simulink model "hexa_tilted_ANSFT"  (R2023a)
settings: Solver=ode1  StartTime=0.0  StopTime=tf  FixedStep=0.01  RelTol=1e-3
model workspace (MAT data in the model file):
  hover_2m = [0  0  0  0  0  0; 0  0  0  0  0  0; 2  2  2  2  2  2; 0  0  0  0  0  0; 0  0  0  0  0  0; 0  0  0  0  0  0]
  square = [0  0  0  0  0  0; 0  0  0  0  0  0; 2.5  2.5  2.5  2.5  2.5  0; 0  0  0  0  0  0; 0  0  0  0  0  0; 0  0  0  0  0  0]
  tf = Simulink.Parameter
  tf.Value = 60
  tf.DataType = 'auto'
  tf.Complexity = 'real'
  tf.Dimensions = [1 1]
  tray0 = [0  0  0  0  0  0; 0  0  0  0  0  0; 0  5  5  5  5  0; 0  0  0  0  0  0; 0  0  0  0  0  0; 0  0  0  0  0  0]
  tray1 = [0  0  0  0  0  0; 0  0  0  0  0  0; 0  5  2.5  5  2.5  0; 0  0  0  0  0  0; 0  0  0  0  0  0; 0  0  0  0  0  0]
  tray2 = [0  2  2  -2  -2  0; 0  0  -2  -2  2  0; 0  5  2.5  5  2.5  0; 0  0  0  0  0  0; 0  0  0  0  0  0; 0  0  0  0  0  0]
  tray3 = [0  2  2  -2  -2  0; 0  0  -2  -2  2  0; 0  5  2.5  5  2.5  0; 0  0  0  0  0  0; 0  0  0  0  0  0; 0  0  0.785  1.57  0.785  0]
  tray4 = [0  2  2  -2  -2  0; 0  0  -2  -2  2  0; 0  5  2.5  5  2.5  0; 0  0.15  0.15  0.15  0.15  0; 0  0  0  0  0  0; 0  0  0.785  1.57  0.785  0]
  tray5 = [0  0  0  0  0  0; 0  0  0  0  0  0; 0  5  2.5  5  2.5  0; 0  0.15  0.15  0  0  0; 0  0  0.15  0.15  0  0; 0  0  0  0  0  0]
  tray_yaw = [0  0  0  0  0  0; 0  0  0  0  0  0; 0  5  2.5  5  2.5  0; 0  0  0  0  0  0; 0  0  0  0  0  0; 0  0  0.785  1.57  0.785  0]
values from neighbouring files (symbols this model uses):
  F = [fx; fy; fz; tx; ty; tz]    [dump_quad_formulas.m]
undefined symbols (not defined in the file or in its folder): Light, MIL, sigbuilder_block
libraries: SignalEditorBlockLib x2, robotcorelib x1, sharedtransform x1, aerolibwind2 x1
settings Model: Creator=adan  LastModifiedBy=Adan Daniel
settings OptimizationCC: DefaultParameterBehavior=Inlined  EnhancedBackFolding=on  PassReuseOutputArgsAs=Individual arguments  ZeroExternalMemoryAtStartup=off  ZeroInternalMemoryAtStartup=off  OptimizeBlockOrder=speed  DifferentSizesBufferReuse=on  OptimizationCustomize=off  EfficientTunableParamExpr=on
settings DebuggingCC: ParameterTunabilityLossMsg=error
settings SFSimCC: MATLABDynamicMemAlloc=off
settings RTWCC: Description=Embedded Coder  SystemTargetFile=ert.tlc  TemplateMakefile=ert_default_tmf
settings CodeAppCC: ForceParamTrailComments=on  IgnoreCustomStorageClasses=off  OperatorAnnotations=on  SimulinkDataObjDesc=on  SFDataObjDesc=on  InsertBlockDesc=on
settings ERTTargetCC: TargetLangStandard=C99 (ISO)  GenerateSampleERTMain=on  InlinedParameterPlacement=NonHierarchical  ERTCustomFileTemplate=example_file_process.tlc

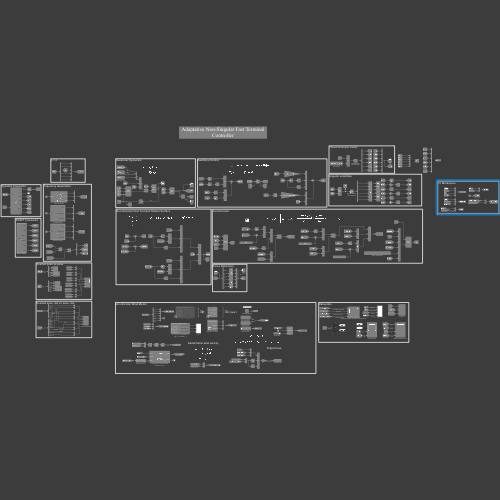
[thumbnail: Simulink's stored preview of the top-level diagram]
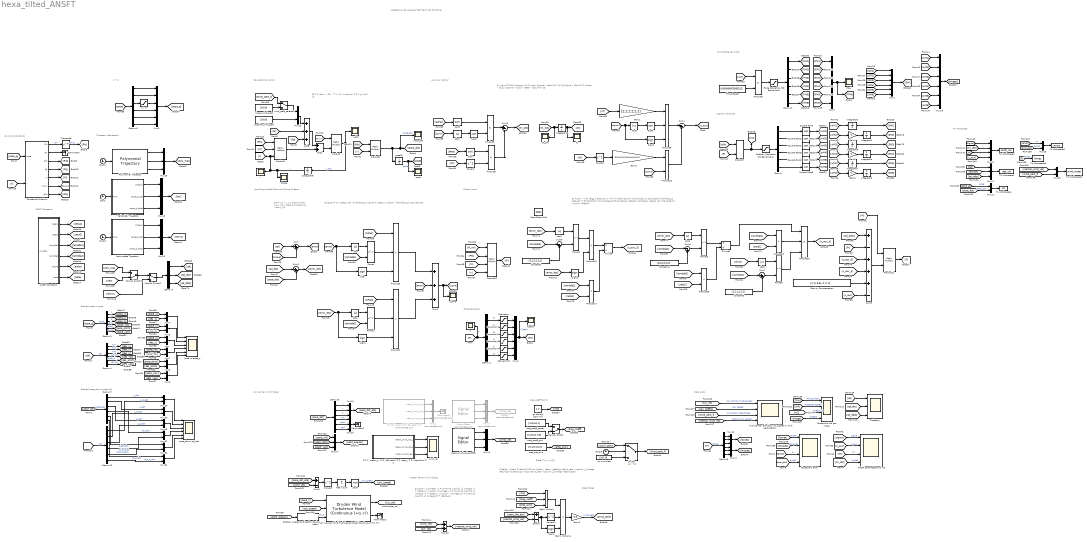
== system hexa_tilted_ANSFT ==
  note: To Workspace
  note: Von Kármán Wind Model
  note: $\Delta _ {\eta} = \frac{1}{2}\rho \alpha _ \eta A _\eta\big (\dot d_\eta - \upsilon _{\omega \eta}\big)^2\text{sign }\big (\dot d_\eta - \upsilon _{\omega \eta}\big)$$
  note: drag coeff from []
  note: $\upsilon _{\omega x} = \overline \upsilon _{ \omega x} + \delta_u \\ \upsilon _{\omega y} = \overline \upsilon _{ \omega y} + \delta_u \\ \upsilon _{\omega z} = \overline \upsilon _{ \omega z} + \delta_u$
  note: Auxiliary Control
  note: Non-Singular Fast Terminal Sliding Surface
  note: Control Input
  note: $e = x_d - x_1 \\ \dot e = \dot x_d - x_2 \\ \ddot e = \ddot x_d - \dot x_2$
  note: z > 0
  note: Adaptative Non-Singular Fast Terminal Controller
  note: ANSFT Constants
  note: Desired pose vs pose
  note: Trajectory Generation
  note: Dynamic Constants
  note: Data plots
  note: Angular velocities
  note: Thrust force per motor
  note: Hexarotor Dynamics
  note: Force Saturation
  note: $u = g(x) ^{-1} \Bigg [ \ddot \chi_d - f(x) + \frac{|\dot e|^{2-\lambda_2} sign(\dot e)}{\lambda_2 \zeta_2} + \frac{|\dot e|^{2-\lambda_2}}{\lambda_2 \zeta_2} \lambda_1 \zeta_1 |e|^{\lambda-1} - u_{aux} \Bigg ]$
  note: $\sigma = e + \zeta_1 |e| ^{\lambda_1} sign(e) + \zeta_2 | \dot e| ^{\lambda_2} sign(\dot e)$
  note: $u_{aux}=-2K(t) |\sigma|^{1/2} sign (\sigma) - \frac{K(t)^2}{2}\sigma \\ \dot K(t) = \alpha ^{1/2} |\sigma| ^{1/2} - \beta ^{1/2}K(t)^2$
  note: $F = M \dot v - \Phi ^T (v) Mv \\ \dot \chi = R^i_b (\chi) v$
  note: $\eta = \{x,y,z\}$
  note: Drag Forces
  note: Inertial frame wind velocity
  note: Desired pose_dot vs pose_dot
  ANSFT Constants : MATLAB Function  TreatAsAtomicUnit=on
  ANSFT parameters and vel : Scope  NumInputPorts=4
  Abs{,1..6} (7 alike) : Abs  SaturateOnIntegerOverflow=off
  Add2 : Sum
  Add5 : Sum  Inputs=+++
  Clock{,1..3} (4 alike) : Clock
  Constant2 : Constant  Value=[2;2;2;2;2;2]
  Constant3 : Constant  Value=[1;1;1;1;1;1]
  Constant4 : Constant  Value=[2;2;2;2;2;2]
  Constants Functions : MATLAB Function  TreatAsAtomicUnit=on
  Demux{,1..6,8..10} (10 alike) : Demux  Outputs=6
  Demux7 : Demux  Outputs=3
  Divide : Product  Inputs=*/
  Divide1 : Product  Inputs=*/
  F : Scope
  F_satur : Scope
  Force Saturation (RC Benchmark) : Saturate  UpperLimit=10  LowerLimit=0
  Forces and Vel per motor : Scope  NumInputPorts=4
  Forces and error : Scope  NumInputPorts=4
  Gain1 : Gain  Gain=[2;2;2;2;2;2]
  Gain2 : Gain  Gain=[0.5;0.5;0.5;0.5;0.5;0.5]
  Gain3 : Gain  Gain=-0.5
  Gain4 : Gain  Gain=-1
  Gain5 : Gain  Gain=-1
  Gain6 : Gain  Gain=-1
  Goto64 : Goto  Commented=on  GotoTag=wind_vel
  Gravity Compensation : Constant  Value=[0; 0; 9.81; 0; 0; 0]
  Helicoidal Trajectory : MATLAB Function  TreatAsAtomicUnit=on
  Integrator2 : Integrator  InitialCondition=[0;0;0;0;0;0]
  Integrator{3..8} (6 alike) : Integrator
  Kt : Scope
  Kt_dot : Scope
  Lemniscate Trajectory : MATLAB Function  TreatAsAtomicUnit=on
  Manual Switch : ManualSwitch  CurrentSetting=0
  Manual Switch1 : ManualSwitch  CurrentSetting=0
  Manual Switch2 : ManualSwitch
  Matrix Sum : Sum  Inputs=+
  Matrix Multiply : Product  Inputs=3
  Matrix Multiply1 : Product  Inputs=3
  Mux{,4..8,13,22..23,25,28..33} (16 alike) : Mux  Inputs=2
  Mux{1..3,9,26} (5 alike) : Mux  Inputs=6
  Mux{10,12,14..16,18..21,27} (10 alike) : Mux  Inputs=3
  Mux11 : Mux  Commented=on  Inputs=3
  Mux17 : Mux  Commented=on  Inputs=3
  Mux24 : Mux
  Polynomial Trajectory : robotcorelib/Polynomial Trajectory  WaypointSource=Internal  Waypoints=hover_2m  TimePoints=[ 0, 12, 24, 36, 48, tf ]  TimeInterval=[ 1, 4 ]  Method=Cubic Polynomial  ParameterSource=Internal  VelocityBoundaryCondition=zeros( 6, 6 )  AccelerationBoundaryCondition=zeros( 2, 5 )  SimulateUsing=Interpreted execution
  Power{,1,4..6} (5 alike) : Math  Operator=pow
  Power{2..3,9,11} (4 alike) : Math  Operator=square
  Product{,2,7,11} (4 alike) : Product  Multiplication=Matrix(*)
  Product1 : Product  Inputs=3  Multiplication=Matrix(*)
  Product{5..6,9..10,13..15,18} (8 alike) : Product
  Product12 : Product  Inputs=4  Multiplication=Matrix(*)
  Product{3..4,8,16} (4 alike) : Product  Inputs=3
  Rotation Angles to Direction Cosine Matrix : sharedtransform/Rotation Angles to Direction Cosine Matrix  rotationOrder=ZYX  aMode=aMode
  Rotation Saturation (RC Benchmark) : Saturate  UpperLimit=818608.7529  LowerLimit=0
  Saturation : Saturate  UpperLimit=6  LowerLimit=-6
  Saturation1 : Saturate  UpperLimit=6  LowerLimit=-6
  Saturation2 : Saturate  UpperLimit=5.8*6  LowerLimit=0
  Saturation3 : Saturate
  Saturation4 : Saturate
  Saturation5 : Saturate
  Scope : Scope
  Sign{,1..4} (5 alike) : Signum
  Signal Editor : SignalEditorBlockLib/Signal Editor  Commented=on  FileName=C:\Users\Adan Daniel\Documents\IMT\8Semestre_tec\Diseño e implementación de sistemas mecatronicos\mean_wind_vel.mat  ActiveScenario=Velocidades_medias_del_viento  ActiveSignal=wean_wind_vel_x  IsBus=off  OutputBusObjectStr=Bus: BusObject  SampleTime=0  Interpolate=off  ZeroCross=off  OutputAfterFinalValue=Setting to zero  Unit=inherit  PreserveSignalName=on  ApplySigPropsToAllScenarios=on
  Sqrt{,1..4} (5 alike) : Sqrt
  Square Root{,1..5} (6 alike) : Sqrt
  Sum{,2..3,7} (4 alike) : Sum  Inputs=|+-
  Sum1 : Sum  Inputs=+++
  Sum13 : Sum
  Sum14 : Sum  Inputs=+-
  Sum4 : Sum  Inputs=|--
  Sum5 : Sum  Inputs=+-+++-
  Sum6 : Sum  Inputs=|-+
  Sum8 : Sum  Inputs=|-+
  Sum9 : Sum  Inputs=+-
  Switch : Switch  Criteria=u2 > Threshold  Threshold=10  SaturateOnIntegerOverflow=off  InputSameDT=off
  TFMi : Scope
  Terminator : Terminator
  Terminator1 : Terminator
  Terminator2 : Terminator
  Terminator3 : Terminator  Commented=on
  Thrust Factor : Constant  Value=0.000006975938113
  To Workspace : ToWorkspace  VariableName=des_chi  SaveFormat=Structure With Time  SampleTime=-1
  To Workspace1 : ToWorkspace  VariableName=chi  SaveFormat=Structure With Time  SampleTime=-1
  To Workspace2 : ToWorkspace  VariableName=errors  SaveFormat=Structure With Time  SampleTime=-1
  To Workspace3 : ToWorkspace  VariableName=forces  SaveFormat=Structure With Time  SampleTime=-1
  To Workspace4 : ToWorkspace  VariableName=ansft_var  SaveFormat=Structure With Time  SampleTime=-1
  To Workspace5 : ToWorkspace  VariableName=wind_model  SaveFormat=Structure With Time  SampleTime=-1
  Trajectory : Scope  NumInputPorts=3
  Transpose : Math  Operator=transpose
  "Turbulence velocities, uav_speed & wind perturbation" : Scope  NumInputPorts=4
  Von Karman Wind Turbulence Model (Continuous (+q +r)) : aerolibwind2/Dryden Wind Turbulence Model  (Continuous (+q -r))  units=Metric (MKS)  spec=MIL-F-8785C  model=Continuous Von Karman (+q -r)  W20=15  Wdeg=0  TurbProb=10^-2 - Light  L_high=762  Wingspan=10  ts=0.1  Seed=[23341 23342 23343 23344]  T_on=on
      settings: LibrarySourceBlock=|
      | aerolibwind2/Von Karman Wind Turbulence Model
      | (Continuous (+q +r))
  Zero-Order Hold : ZeroOrderHold  SampleTime=-1
  air density [kg/m^3] : Constant  Value=1.2
  angular_wind_perb : Constant  Value=[0;0;0]
  area_per_axis : Constant  Value=[0.1;0.1;0.2]
  drag_coeff_gus : Constant  Value=[0.3;0.3; 0.5]
  drag_coeff_paper : Constant  Value=[0.6;0.6; 1]
  f = 1 | mean_xy = 5 | deviation = 2 mea_y = 3 | devaition = 2 : Subsystem  Tag=STV Subsys  LoadFcn=sigbuilder_block('load');  StartFcn=sigbuilder_block('start');  StopFcn=sigbuilder_block('stop');  ClipboardFcn=sigbuilder_block('clipboard');  mask(Sigbuilder block){tuvar=[0:10]}
      mask help: Simulink:masks:SigbuilderBlock_MD
      mask init:
      | if ~strcmp(get_param(bdroot(gcbh),'SimulationStatus'),'stopped') tuvar = sigbuilder_block('maskInit'); end
      settings: CopyFcn=sigbuilder_block('copy');  DeleteFcn=sigbuilder_block('delete');  ModelCloseFcn=sigbuilder_block('modelClose');  PreSaveFcn=sigbuilder_block('preSave');  PauseFcn=sigbuilder_block('pause');  ContinueFcn=sigbuilder_block('continue');  NameChangeFcn=sigbuilder_block('namechange');  OpenFcn=sigbuilder_block('open',[0 0 1024.5 518.25 ]);  CloseFcn=sigbuilder_block('close');
      mask Display: plot(0, 0, 100, 100,[2, 2, 32, 32, 2], [68, 8, 8, 68, 68],[32, 2], [38, 38], [32, 19, 2],[53, 60, 44], [32, 17, 17, 2],[16, 16, 31, 31]);txt = getActiveGroup(gcbh);text(2, 100, txt,'verticalAlignment', 'top');
  f = 10 | mean = 3 | deviation = 1 : Subsystem  Tag=STV Subsys  Commented=on  LoadFcn=sigbuilder_block('load');  StartFcn=sigbuilder_block('start');  StopFcn=sigbuilder_block('stop');  ClipboardFcn=sigbuilder_block('clipboard');  mask(Sigbuilder block){tuvar=[0:10]}
      mask help: Simulink:masks:SigbuilderBlock_MD
      mask init:
      | if ~strcmp(get_param(bdroot(gcbh),'SimulationStatus'),'stopped') tuvar = sigbuilder_block('maskInit'); end
      settings: CopyFcn=sigbuilder_block('copy');  DeleteFcn=sigbuilder_block('delete');  ModelCloseFcn=sigbuilder_block('modelClose');  PreSaveFcn=sigbuilder_block('preSave');  PauseFcn=sigbuilder_block('pause');  ContinueFcn=sigbuilder_block('continue');  NameChangeFcn=sigbuilder_block('namechange');  OpenFcn=sigbuilder_block('open',[6 0 1012.5 477.75 ]);  CloseFcn=sigbuilder_block('close');
      mask Display: plot(0, 0, 100, 100,[2, 2, 32, 32, 2], [68, 8, 8, 68, 68],[32, 2], [38, 38], [32, 19, 2],[53, 60, 44], [32, 17, 17, 2],[16, 16, 31, 31]);txt = getActiveGroup(gcbh);text(2, 100, txt,'verticalAlignment', 'top');
  linear_wind_perb : Constant  Value=[0;0;0]
  mean_wind_vel_ansft[1] : SignalEditorBlockLib/Signal Editor  FileName=C:\Users\Adan Daniel\Documents\IMT\8Semestre_tec\Diseño e implementación de sistemas mecatronicos\mean_wind_vel_ansft.mat  ActiveScenario=Velocidades_medias_del_viento  ActiveSignal=wean_wind_vel_x  IsBus=off  OutputBusObjectStr=Bus: BusObject  SampleTime=0  Interpolate=off  ZeroCross=off  OutputAfterFinalValue=Setting to zero  Unit=inherit  PreserveSignalName=on  ApplySigPropsToAllScenarios=on
  no wind perb : Constant  Value=[0;0; 0]
  pose : Scope
  pose vs pose_q : Scope  NumInputPorts=6
  pose(0) : Integrator  InitialCondition=[2; 0; 0; 0; 0; 0]
  pose_dot : Scope
  pose_dot vs qd_dot : Scope  NumInputPorts=6
  pose_dot(0) : Integrator  InitialCondition=[0; 0; 0; 0; 0; 0]
  sigma : Scope
  v : Scope
  v_dot : Scope
  wind vel : Scope  NumInputPorts=3
  wind_perb_selector : ManualSwitch
  z > 0 : Saturate  UpperLimit=100  LowerLimit=0
  wires:
  Saturation/1 -> Mux2/1
  Saturation1/1 -> Mux2/2
  Saturation4/1 -> Mux2/5
  Saturation3/1 -> Mux2/4
  Demux1/6 -> Saturation5/1  "tz"
  Demux1/3 -> Saturation2/1  "Fz"
  [F] -> F/1, Demux1/1  "F"
  Saturation5/1 -> Mux2/6
  Demux1/2 -> Saturation1/1  "Fy"
  Demux1/1 -> Saturation/1  "Fx"
  Demux1/5 -> Saturation4/1  "ty"
  Demux1/4 -> Saturation3/1  "tx"
  Saturation2/1 -> Mux2/3
  Mux2/1 -> [F2], F_satur/1  "F_satur"
  [M] -> Product1/2
  [v] -> Product2/2
  [M_inv] -> Product/1
  Add2/1 -> Product/2
  Product/1 -> v_dot/1, pose_dot(0)/1  "v_dot"
  [Rib] -> Product2/1
  Product2/1 -> pose(0)/1, pose_dot/1, [pose_dot]  "pose_dot"
  [Phi] -> Product1/1
  Product1/1 -> Add2/2
  pose(0)/1 -> pose/1, [pose]  "pose"
  pose_dot(0)/1 -> Scope/1, v/1, [v], Product1/3  "v"
  [Fg] -> Add5/3
  Add5/1 -> Add2/1
  [FM6] -> Mux3/6
  Demux2/2 -> [FM2]
  [FM3] -> Mux3/3
  Demux2/6 -> [FM6]
  [FM5] -> Mux3/5
  Force Saturation (RC Benchmark)/1 -> Demux2/1
  [FM2] -> Mux3/2
  [FM1] -> Mux3/1
  Demux2/5 -> [FM5]
  Demux2/4 -> [FM4]
  Product9/1 -> Force Saturation (RC Benchmark)/1
  Demux2/1 -> [FM1]
  Thrust Factor/1 -> Product9/2
  Demux2/3 -> [FM3]
  [w2] -> Product9/1
  [FM4] -> Mux3/4
  [wM1] -> Integrator3/1
  Square Root/1 -> [wM1]
  [wM5] -> Integrator7/1
  Square Root5/1 -> [wM6]
  Square Root3/1 -> [wM4]
  [F] -> Product7/2
  [allo] -> Product7/1
  [wM2] -> Gain4/1
  Demux/6 -> Square Root5/1
  Demux/5 -> Square Root4/1
  Square Root1/1 -> [wM2]
  [wM3] -> Integrator5/1
  Square Root2/1 -> [wM3]
  Demux/4 -> Square Root3/1
  Demux/2 -> Square Root1/1
  Demux/3 -> Square Root2/1
  Square Root4/1 -> [wM5]
  Product7/1 -> [w2], Rotation Saturation (RC Benchmark)/1
  Demux/1 -> Square Root/1
  [wM4] -> Gain5/1
  [wM6] -> Gain6/1
  Mux3/1 -> [TFMi], TFMi/1
  [u_aux] -> ANSFT parameters and vel/2  "u_aux"
  [sigma] -> ANSFT parameters and vel/1  "sigma"
  [Kt_dot] -> ANSFT parameters and vel/4  "Kt_dot"
  [pose_g] -> Constants Functions/1(pose)
  [v] -> Constants Functions/2(v)
  Constants Functions/7(allo) -> [allo]
  Constants Functions/4(Fg) -> [Fg]
  Constants Functions/5(M) -> [M]
  Constants Functions/1(Phi) -> Transpose/1  "phi"
  Constants Functions/3(Rib) -> [Rib]
  Transpose/1 -> [Phi]  "phi_T"
  Constants Functions/6(M_inv) -> [M_inv]
  Clock1/1 -> Polynomial Trajectory/1
  Polynomial Trajectory/3 -> Mux19/3
  Mux/1 -> pose vs pose_q/3
  [qd] -> Demux4/1  "qd"
  [pose_g] -> Demux3/1  "pose"
  Mux5/1 -> pose vs pose_q/2
  Mux4/1 -> pose vs pose_q/1
  Polynomial Trajectory/1 -> Mux19/1
  [error] -> Forces and error/3  "e"
  [error_dot] -> Forces and error/4  "e_dot"
  Mux6/1 -> pose vs pose_q/6
  Mux7/1 -> pose vs pose_q/4
  Mux8/1 -> pose vs pose_q/5
  [Kt] -> ANSFT parameters and vel/3  "Kt"
  Demux5/5 -> Mux9/5
  Demux5/6 -> Mux9/6
  Mux9/1 -> [pose_g]
  Demux5/1 -> Mux9/1
  Demux5/3 -> z > 0/1
  Demux5/2 -> Mux9/2
  Demux5/4 -> Mux9/4
  [pose] -> Demux5/1
  z > 0/1 -> Mux9/3
  ANSFT Constants/3(lambda1) -> [lambda1]
  ANSFT Constants/1(zeta1) -> [zeta1]
  ANSFT Constants/2(zeta2) -> [zeta2]
  ANSFT Constants/4(lambda2) -> [lambda2]
  ANSFT Constants/5(alpha) -> [alpha]
  ANSFT Constants/6(beta) -> [beta]
  Product16/1 -> [u_aux_4]
  [error_dot] -> Sign3/1
  Product15/1 -> Product16/2
  [error_dot] -> Abs4/1
  [u_aux_4] -> Sum5/4
  [lambda1] -> Sum7/1
  [error] -> Abs5/1
  Abs5/1 -> Power5/1
  Sign3/1 -> Product13/2
  [qd_ddot] -> Sum5/1
  [lambda2] -> Product14/1
  Constant2/1 -> Sum6/2
  [Phi] -> Product12/2
  Constant3/1 -> Sum7/2
  [u_aux] -> Sum5/6
  Product13/1 -> Divide/1
  [M] -> Product11/1
  [u_aux_3] -> Sum5/3
  Divide/1 -> [u_aux_3]
  Sum5/1 -> Product11/2
  Sum6/1 -> Power4/2
  Sum7/1 -> Power5/2
  [zeta1] -> Product15/2
  Product14/1 -> Divide/2
  [fx] -> Sum5/2
  [v] -> Product12/4
  Power5/1 -> Product16/3
  Abs4/1 -> Power4/1
  [M] -> Product12/3
  Product12/1 -> [fx]
  [lambda1] -> Product15/1
  [M_inv] -> Product12/1
  [zeta2] -> Product14/2
  [lambda2] -> Sum6/1
  Power4/1 -> Product13/1
  Product11/1 -> [F]
  Sign/1 -> Product3/3
  [lambda1] -> Power/2
  [qd_dot] -> Sum2/1
  Power1/1 -> Product4/2
  Abs/1 -> Power/1
  [pose_dot] -> Sum2/2
  Abs1/1 -> Power1/1
  [zeta1] -> Product3/1
  Power/1 -> Product3/2
  [error_dot] -> Sign1/1, Abs1/1
  [lambda2] -> Power1/2
  [zeta2] -> Product4/1
  Product4/1 -> Sum1/3
  Sum/1 -> [error]
  Sum2/1 -> [error_dot]
  Product3/1 -> Sum1/1
  Sum1/1 -> sigma/1, [sigma]
  [error] -> Sign/1, Abs/1
  [qd] -> Sum/1
  [pose_g] -> Sum/2
  Sign1/1 -> Product4/3
  [error] -> Sum1/2
  Gain2/1 -> Product10/1
  Product6/1 -> Sum3/2
  Sum4/1 -> [u_aux]
  Integrator2/1 -> Kt/1, [Kt]
  [Kt] -> Power2/1
  Sqrt2/1 -> Product5/2
  [beta] -> Sqrt/1
  Abs2/1 -> Sqrt2/1
  Product8/1 -> Sum4/1
  Sqrt3/1 -> Product8/2
  Product5/1 -> Sum3/1
  [sigma] -> Sign2/1, Abs3/1
  [sigma] -> Product10/2
  Sqrt/1 -> Product6/1
  Sign2/1 -> Product8/3
  Sqrt1/1 -> Product5/1
  [Kt_dot] -> Kt_dot/1, Integrator2/1
  Product10/1 -> Sum4/2
  [Kt] -> Power3/1
  Sum3/1 -> [Kt_dot]
  Power3/1 -> Gain2/1
  [sigma] -> Abs2/1
  [Kt] -> Gain1/1
  Gain1/1 -> Product8/1
  Abs3/1 -> Sqrt3/1
  [alpha] -> Sqrt1/1
  Power2/1 -> Product6/2
  Divide1/1 -> Product16/1
  [lambda2] -> Sum8/1
  Product18/1 -> Divide1/2
  Power6/1 -> Divide1/1
  [lambda2] -> Product18/1
  Sum8/1 -> Power6/2
  [zeta2] -> Product18/2
  Constant4/1 -> Sum8/2
  [error_dot] -> Abs6/1
  Abs6/1 -> Power6/1
  Gravity Compensation/1 -> Sum5/5
  [F2] -> Add5/2
  Demux3/1 -> [pose_x]  "x"
  Demux3/2 -> [pose_y]  "y"
  Demux3/3 -> [pose_z]  "z"
  Demux3/4 -> [pose_roll]  "roll"
  Demux3/6 -> [pose_yaw]  "yaw"
  Demux3/5 -> [pose_pitch]  "pitch"
  Demux4/6 -> [des_yaw]  "yaw_d"
  Demux4/5 -> [des_pitch]  "pitch_d"
  Demux4/3 -> [des_z]  "z_d"
  Demux4/1 -> [des_x]  "x_d"
  Demux4/4 -> [des_roll]  "roll_d"
  Demux4/2 -> [des_y]  "y_d"
  [pose_x] -> Mux4/1
  [des_x] -> Mux4/2
  [pose_y] -> Mux5/1
  [pose_z] -> Mux/1
  [pose_roll] -> Mux7/1
  [pose_pitch] -> Mux8/1
  [pose_yaw] -> Mux6/1
  [des_y] -> Mux5/2
  [des_z] -> Mux/2
  [des_roll] -> Mux7/2
  [des_pitch] -> Mux8/2
  [des_yaw] -> Mux6/2
  [pose_z] -> Von Karman Wind Turbulence Model (Continuous (+q +r))/1
  Constants Functions/2(R1) -> Terminator/1
  [pose_dot] -> Demux6/1
  Demux6/1 -> Mux16/1  "x"
  Demux6/2 -> Mux16/2  "y"
  Demux6/3 -> Mux16/3  "z"
  Demux6/4 -> Mux10/1  "roll"
  Demux6/5 -> Mux10/2  "pitch"
  Demux6/6 -> Mux10/3  "yaw"
  Power9/1 -> Matrix Sum/1
  Matrix Sum/1 -> Sqrt4/1
  Sqrt4/1 -> [uav_speed]  "uav_speed"
  Von Karman Wind Turbulence Model (Continuous (+q +r))/1 -> [tur_vel]
  Von Karman Wind Turbulence Model (Continuous (+q +r))/2 -> Terminator1/1
  Rotation Angles to Direction Cosine Matrix/1 -> Von Karman Wind Turbulence Model (Continuous (+q +r))/3  "phi_T"
  [uav_speed] -> Von Karman Wind Turbulence Model (Continuous (+q +r))/2
  air density [kg/m^3]/1 -> [rho]
  area_per_axis/1 -> [area_axis]
  Gain3/1 -> [Wind_perb]  "wind_perb"
  [rho] -> Matrix Multiply/1
  [drag_coeff] -> Matrix Multiply/2
  [area_axis] -> Matrix Multiply/3
  Power11/1 -> Matrix Multiply1/2
  Matrix Multiply/1 -> Matrix Multiply1/1
  Matrix Multiply1/1 -> Gain3/1
  Sum14/1 -> Sign4/1, Power11/1
  Sign4/1 -> Matrix Multiply1/3
  angular_wind_perb/1 -> Mux13/2
  Mux13/1 -> Add5/1
  linear_wind_perb/1 -> wind_perb_selector/2
  [Wind_perb_f] -> wind_perb_selector/1
  wind_perb_selector/1 -> Mux13/1
  Mux10/1 -> Terminator2/1
  [pose_angular] -> Rotation Angles to Direction Cosine Matrix/1
  Mux14/1 -> [pose_angular]
  [pose_yaw] -> Mux14/3
  [pose_pitch] -> Mux14/2
  [pose_roll] -> Mux14/1
  [wind_vel] -> Sum13/1
  Mux16/1 -> [pose_dot_eta]
  Sum13/1 -> [inertial_wind_vel]
  [tur_vel] -> Sum13/2
  [pose_dot_eta] -> Sum14/1
  [inertial_wind_vel] -> Sum14/2
  f = 10 | mean = 3 | deviation = 1/2(wean_wind_vel_y) -> Mux11/2
  f = 10 | mean = 3 | deviation = 1/1(wean_wind_vel_x) -> Mux11/1
  f = 10 | mean = 3 | deviation = 1/3(wean_wind_vel_z) -> Mux11/3
  [pose_dot_eta] -> Sum9/1
  Sum9/1 -> Power9/1
  [wind_vel] -> Sum9/2
  [Wind_perb_f] -> "Turbulence velocities, uav_speed & wind perturbation"/3  "wind perb | drag forces"
  [inertial_wind_vel] -> "Turbulence velocities, uav_speed & wind perturbation"/4  "inertia wind velocity"
  [tur_vel] -> "Turbulence velocities, uav_speed & wind perturbation"/1  "Von Kármán Turbulences"
  [uav_speed] -> "Turbulence velocities, uav_speed & wind perturbation"/2  "UAV speed"
  Manual Switch/1 -> [drag_coeff]
  drag_coeff_paper/1 -> Manual Switch/1
  drag_coeff_gus/1 -> Manual Switch/2
  Signal Editor/3 -> Mux17/3
  Signal Editor/2 -> Mux17/2
  Signal Editor/1 -> Mux17/1
  Mux17/1 -> Goto64/1
  Mux11/1 -> Terminator3/1
  mean_wind_vel_ansft[1]/2 -> Mux15/2
  Mux15/1 -> [wind_vel]
  mean_wind_vel_ansft[1]/3 -> Mux15/3
  Clock/1 -> Helicoidal Trajectory/1(time)
  Polynomial Trajectory/2 -> Mux19/2
  Mux19/1 -> [poly_traj]
  Mux18/1 -> [heli]
  Helicoidal Trajectory/1(pose_d) -> Mux18/1
  Helicoidal Trajectory/2(pose_d_dot) -> Mux18/2
  Helicoidal Trajectory/3(pose_d_ddot) -> Mux18/3
  [poly_traj] -> Manual Switch1/1
  [heli] -> Manual Switch1/2
  Demux7/1 -> [qd]
  Demux7/2 -> [qd_dot]
  Demux7/3 -> [qd_ddot]
  [qd] -> Trajectory/1
  [qd_dot] -> Trajectory/2
  [qd_ddot] -> Trajectory/3
  Lemniscate Trajectory/2(pose_d_dot) -> Mux20/2
  Clock2/1 -> Lemniscate Trajectory/1(time)
  Lemniscate Trajectory/3(pose_d_ddot) -> Mux20/3
  Mux20/1 -> [lemni]
  Lemniscate Trajectory/1(pose_d) -> Mux20/1
  [lemni] -> Manual Switch2/2
  Manual Switch1/1 -> Manual Switch2/1
  Manual Switch2/1 -> Demux7/1
  [Wind_perb] -> Switch/1
  Clock3/1 -> Switch/2
  no wind perb/1 -> Switch/3
  Switch/1 -> [Wind_perb_f]
  Gain4/1 -> Integrator4/1
  Gain5/1 -> Integrator6/1
  Gain6/1 -> Integrator8/1
  Integrator4/1 -> [SM2]
  Integrator5/1 -> [SM3]
  Integrator7/1 -> [SM5]
  Integrator3/1 -> [SM1]
  Integrator6/1 -> [SM4]
  Integrator8/1 -> [SM6]
  [SM1] -> Mux1/1
  [SM2] -> Mux1/2
  [SM3] -> Mux1/3
  [SM4] -> Mux1/4
  [SM5] -> Mux1/5
  [SM6] -> Mux1/6
  Mux1/1 -> [SMi]
  Rotation Saturation (RC Benchmark)/1 -> Demux/1
  mean_wind_vel_ansft[1]/1 -> Mux15/1
  [qd_dot] -> Mux21/2
  [qd] -> Mux21/1
  [qd_ddot] -> Mux21/3
  Mux21/1 -> To Workspace/1
  [pose_dot] -> Mux22/2  "pose_dot"
  [pose_g] -> Mux22/1  "pose"
  Mux22/1 -> To Workspace1/1
  [error] -> Mux23/1  "e"
  [error_dot] -> Mux23/2  "e_dot"
  Mux23/1 -> To Workspace2/1
  [F] -> To Workspace3/1  "forces"
  [sigma] -> Mux24/1
  [Kt_dot] -> Mux24/2
  [Kt] -> Mux24/3
  [u_aux] -> Mux24/4
  Mux24/1 -> To Workspace4/1
  [SMi] -> Forces and Vel per motor/2  "Propeller Speed"
  [TFMi] -> Forces and Vel per motor/1  "Thrust force"
  [w2] -> Forces and Vel per motor/3  "omega^2"
  [inertial_wind_vel] -> Mux25/1
  [Wind_perb_f] -> Mux25/2
  Mux25/1 -> To Workspace5/1
  [wM6] -> Mux26/6
  [wM2] -> Mux26/2
  [wM4] -> Mux26/4
  [wM1] -> Mux26/1
  [wM5] -> Mux26/5
  [wM3] -> Mux26/3
  Mux26/1 -> [omega]
  [omega] -> Forces and Vel per motor/4  "omega"
  f = 1 | mean_xy = 5 | deviation = 2 mea_y = 3 | devaition = 2/1(mean_wind_vel_x) -> wind vel/1
  f = 1 | mean_xy = 5 | deviation = 2 mea_y = 3 | devaition = 2/2(mean_wind_vel_y) -> wind vel/2
  f = 1 | mean_xy = 5 | deviation = 2 mea_y = 3 | devaition = 2/3(mean_wind_vel_z) -> wind vel/3
  [forces] -> Forces and error/1  "Forces"
  [torques] -> Forces and error/2  "Torques"
  [F] -> Demux8/1  "forces"
  Demux8/1 -> Mux12/1
  Demux8/2 -> Mux12/2
  Demux8/3 -> Mux12/3
  Demux8/4 -> Mux27/1
  Demux8/5 -> Mux27/2
  Demux8/6 -> Mux27/3
  Mux12/1 -> [forces]
  Mux27/1 -> [torques]
  [qd_dot] -> Demux10/1  "qd"
  [pose_dot] -> Demux9/1  "pose_dot"
  Mux29/1 -> pose_dot vs qd_dot/1
  Mux32/1 -> pose_dot vs qd_dot/4
  Mux28/1 -> pose_dot vs qd_dot/3
  Mux30/1 -> pose_dot vs qd_dot/2
  Mux33/1 -> pose_dot vs qd_dot/5
  Mux31/1 -> pose_dot vs qd_dot/6
  Demux9/1 -> Mux29/1  "x_dot"
  Demux10/1 -> Mux29/2  "x_d_dot"
  Demux9/2 -> Mux30/1  "y_dot"
  Demux10/2 -> Mux30/2  "y_d_dot"
  Demux9/3 -> Mux28/1  "z_dot"
  Demux10/3 -> Mux28/2  "z_d_dot"
  Demux9/4 -> Mux32/1  "roll_dot"
  Demux9/5 -> Mux33/1  "pitch_dot"
  Demux9/6 -> Mux31/1  "yaw_dot"
  Demux10/4 -> Mux32/2  "roll_d_dot"
  Demux10/5 -> Mux33/2  "pitch_d_dot"
  Demux10/6 -> Mux31/2  "yaw_d_dot"

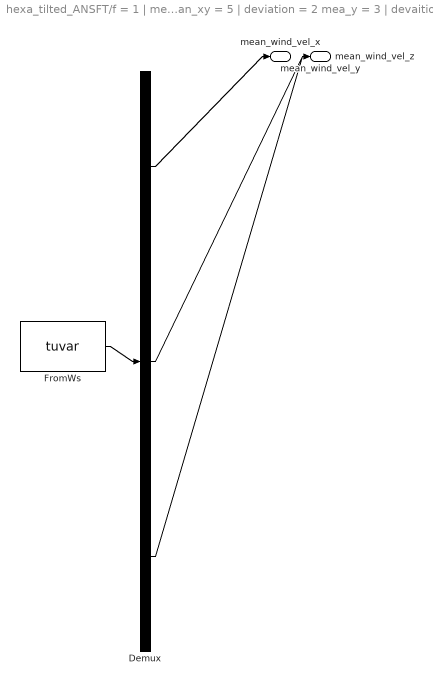
== system hexa_tilted_ANSFT/f = 1 | mean_xy = 5 | deviation = 2 mea_y = 3 | devaition = 2 ==
  Demux : Demux  Tag=STV Demux  Outputs=3
      settings: DisplayOption=none
  FromWs : FromWorkspace  Tag=STV FromWs  VariableName=tuvar  SampleTime=tf
      SigBuilderData=|
      | common.afterFinalStr = 'Extrapolate'
      | common.sampleTime = 'tf'
      | dataSet.timeRange = [0 60]
      | dataSet.name = 'Velocidades medias del viento'
      | sbobj.Groups.Name = 'Velocidades medias del viento'
      | sbobj.Groups.Signals(1).Name = 'mean_wind_vel_x'
      | sbobj.Groups.Signals(1).XData = [0 1 2 3 4 4 5 5 6 7 8 9 10 11 12 13 14 15 16 17 18 19 20 21 22 23 24 25 26 27 28 29 30 31 32 33 34 35 36 37 38 39 40 41 42 43 44 45 46 47 48 49 50 51 52 53 54 55 56 57 58 59 60]
      | sbobj.Groups.Signals(1).YData = [6.07533427909 8.66777002919 0.482306277993 6.72434664074 5.63753047972 5.7 2.4 2.38462340739 4.13281595539 5.68524893308 12.1567938795 10.5388740598 2.30022611969 11.0698469327 6.45080844989 4.87389025362 6.42948580765 4.5900678834 4.75171130357 7.97939521557 7.8180689796 7.83438482686 6.34299426722 2.58502615463 6.43447730266 8.26047057833 5.97778754062 7.06938601984 6.45377026677 4.39311815043 5.58774293419 3.42543439248 6.77679126352 2.70585978606 2.86225908366 3.38100261115 -0.88856832399 7.87676058563 5.65038107891 3.49014336166 7.74059708019 1.57696716229 4.79551510783 4.51710591679 5.63841347833 5.62571719327 3.27024016535 4.93989740761 4.67024196158 6.25541457506 7.18653133808 7.21854659523 3.27269435602 5.15471818226 2.57176591277 2.77299851703 4.98630134379 8.06526061657 3.46066817249 5.74275762552 4.54883119546 7.23471227763 2.8218714099]
      | sbobj.Groups.Signals(2).Name = 'mean_wind_vel_y'
      | sbobj.Groups.Signals(2).XData = [0 1 2 3 4 4 5 5 6 7 8 9 10 11 12 13 14 15 16 17 18 19 20 21 22 23 24 25 26 27 28 29 30 31 32 33 34 35 36 37 38 39 40 41 42 43 44 45 46 47 48 49 50 51 52 53 54 55 56 57 58 59 60]
      | sbobj.Groups.Signals(2).YData = [5.06511492833 6.10505404222 7.20122043576 8.08842379101 5.17186226635 5.2 2.05 2.01681937872 3.51539632548 2.87683653336 9.700914448 3.76879623707 6.49615356741 4.61516297882 6.77722085084 3.47030152686 2.19546206132 2.15524814982 5.97638781972 4.64524968676 4.60789302439 7.83862030129 5.58316874797 5.39562210693 8.17539817995 3.3910680873 6.3932488317 6.67017633015 4.51256971924 5.43134017281 2.66831213704 2.7040944422 5.20974943203 6.44450806445 10.1709825052 3.6662186586 5.37466204916 4.83501114926 1.1339541643 4.12206769213 1.41064231709 6.68075105951 3.22393583534 5.20018566628 3.91094214002 5.6070415893 3.79934687573 5.97993064235 6.47872624721 8.42377556596 4.61175292848 0.72328946112 3.32082250533 7.70918865601 2.85568942323 6.92190773948 5.24809960001 7.87339324544 1.07820000127 4.60460354805 2.58430902948 10.8160160615 6.65043778846]
      | sbobj.Groups.Signals(3).Name = 'mean_wind_vel_z'
      | sbobj.Groups.Signals(3).XData = [0 1 2 3 4 5 6 7 8 9 10 11 12 13 14 15 16 17 18 19 20 21 22 23 24 25 26 27 28 29 30 31 32 33 34 35 36 37 38 39 40 41 42 43 44 45 46 47 48 49 50 51 52 53 54 55 56 57 58 59 60]
      | sbobj.Groups.Signals(3).YData = [5.75794395583 0.883639484025 2.0627688378 2.4550611815 5.19684923578 2.44425613442 4.40308291633 -1.10363259982 2.29230000445 1.35282694969 -0.154114045598 4.01594930181 3.56396812734 3.06695976449 0.332644113144 5.25498455668 3.70035882121 2.40186793933 3.0457795855 2.47600913007 -0.500424736894 2.42869805681 1.33726697686 1.04158738967 0.687196688672 1.93288578137 -1.00527147177 4.92845884526 4.04012020291 2.95994429671 2.93045782794 1.40367283087 5.03737056426 2.73356504098 1.57093967243 5.70277153685 2.55045788789 1.82194193856 2.41249280453 1.30414751272 0.759743397513 8.05199938424 6.31099518577 3.61507031848 0.485763281296 1.26906393889 2.64693177154 4.58283212326 0.33599115737 -1.65973431161 0.101805414323 3.66702166613 3.78270720887 3.90335883786 2.73943069371 3.36737819172 2.04769396676 4.72404322311 0.276611058258 3.91005911289 1.30258124013]
      | sbobj.Groups.TimeRange = [0 60]
  mean_wind_vel_x : Outport  Tag=STV Outport
  mean_wind_vel_y : Outport  Tag=STV Outport  Port=2
  mean_wind_vel_z : Outport  Tag=STV Outport  Port=3
  wires:
  Demux/1 -> mean_wind_vel_x/1
  Demux/2 -> mean_wind_vel_y/1
  Demux/3 -> mean_wind_vel_z/1
  FromWs/1 -> Demux/1

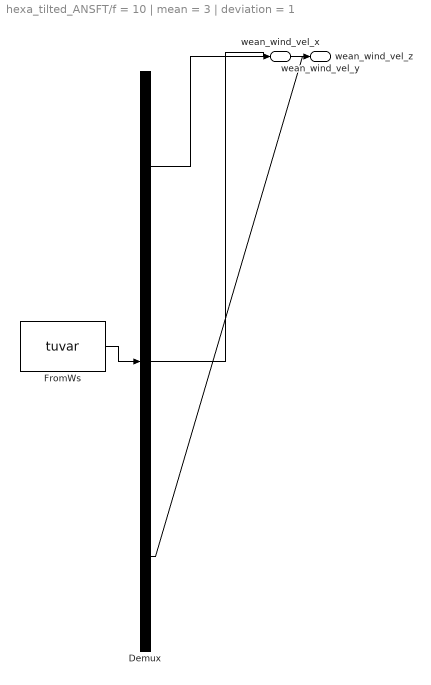
== system hexa_tilted_ANSFT/f = 10 | mean = 3 | deviation = 1 ==
  Demux : Demux  Tag=STV Demux  Outputs=3
      settings: DisplayOption=none
  FromWs : FromWorkspace  Tag=STV FromWs  VariableName=tuvar  SampleTime=tf
      SigBuilderData=|
      | common.afterFinalStr = 'Extrapolate'
      | common.sampleTime = 'tf'
      | dataSet.timeRange = [0 60]
      | dataSet.name = 'Velocidades medias del viento'
      | sbobj.Groups.Name = 'Velocidades medias del viento'
      | sbobj.Groups.Signals(1).Name = 'wean_wind_vel_x'
      | sbobj.Groups.Signals(1).XData = [0 0.1 0.2 0.3 0.4 0.5 0.6 0.7 0.8 0.9 1 1.1 ... (601 elements, 1x601)]
      | sbobj.Groups.Signals(1).YData = [5.53766713955 6.8338850146 2.741153139 5.86217332037 5.31876523986 3.69231170369 4.56640797769 5.34262446654 8.57839693973 7.76943702988 3.65011305984 8.03492346633 ... (601 elements, 1x601)]
      | sbobj.Groups.Signals(2).Name = 'wean_wind_vel_y'
      | sbobj.Groups.Signals(2).XData = [0 0.1 0.2 0.3 0.4 0.5 0.6 0.7 0.8 0.9 1 1.1 ... (601 elements, 1x601)]
      | sbobj.Groups.Signals(2).YData = [5.91223268644 4.52260848431 4.45213058978 6.20133465427 3.99028828723 4.49714503986 5.41986707981 4.64980873263 5.90493344568 5.53412153957 4.79157028877 3.72230146169 ... (601 elements, 1x601)]
      | sbobj.Groups.Signals(3).Name = 'wean_wind_vel_z'
      | sbobj.Groups.Signals(3).XData = [0 0.1 0.2 0.3 0.4 0.5 0.6 0.7 0.8 0.9 1 1.1 ... (601 elements, 1x601)]
      | sbobj.Groups.Signals(3).YData = [6.61794268764 4.42556339349 3.34825928008 4.18131819243 5.7345009623 5.85592925649 4.96022727675 5.08740032024 5.43290557704 3.34095813092 4.21829027453 2.9698506779 ... (601 elements, 1x601)]
      | sbobj.Groups.TimeRange = [0 60]
  wean_wind_vel_x : Outport  Tag=STV Outport
  wean_wind_vel_y : Outport  Tag=STV Outport  Port=2
  wean_wind_vel_z : Outport  Tag=STV Outport  Port=3
  wires:
  FromWs/1 -> Demux/1
  Demux/1 -> wean_wind_vel_x/1
  Demux/2 -> wean_wind_vel_y/1
  Demux/3 -> wean_wind_vel_z/1

== matlab function hexa_tilted_ANSFT/Helicoidal Trajectory ==
  data: time input; pose_d output; pose_d_dot output; pose_d_ddot output
function [pose_d, pose_d_dot, pose_d_ddot]= fcn(time)

pos_z = time / 12;
f = 0.15;
arg = f * (time - 5);
r = 2;

% hover for 5 s | include inclination in roll
% 5 metros al menos

if (time < 5)
    pos_x = 2;
    pos_y = 0;
    roll = 0;
else
    pos_x = r * cos (arg);
    pos_y = r * sin (arg);
    roll = 0.15;
end

% roll = 0;
yaw = time * 0;

pose_d = [pos_x;
          pos_y;
          pos_z;
          roll;
          0;
          yaw];

pos_z_dot = 1 / 12;

% hover for 5 s
if (time < 5)
    pos_x_dot = 0;
    pos_y_dot = 0;
else
    pos_x_dot = - f * r * sin(arg);
    pos_y_dot = f * r * cos(arg);
end

yaw_dot = 0;

pose_d_dot = [pos_x_dot;
              pos_y_dot;
              pos_z_dot;
              0;
              0;
              yaw_dot];

pos_z_ddot = 0;
% hover for 5 s
if (time < 5)
    pos_x_ddot = 0;
    pos_y_ddot = 0;
else
    pos_x_ddot = - f * f * r * cos(arg);
    pos_y_ddot = - f * f * r * sin(arg);
end

yaw_ddot = 0;

pose_d_ddot = [pos_x_ddot;
               pos_y_ddot;
               pos_z_ddot;
               0;
               0;
               yaw_ddot];

== matlab function hexa_tilted_ANSFT/ANSFT Constants ==
  data: unused input; zeta1 output; zeta2 output; lambda1 output; lambda2 output; alpha output; beta output
function [zeta1, zeta2, lambda1, lambda2, alpha, beta] = fcn(~)

%% Constantes de la Superficie deslizante
% valores de zeta1 y zeta2
% zeta1 parecido a una ganancia proporcional
zeta1 = [1.25; 1.25; 0.1; 1; 1; 5];

%zeta2 parecido a una ganancia derivatida
zeta2 = [3; 3; 2; 0.5; 0.5; 0.5];

% lambda 1 > lambda2
lambda1 = [2; 2; 2; 5; 5; 5];

% 1 < lambda2 < 2
lambda2 = [1.6; 1.6; 1.5; 1.5; 1.5; 1.5];

%% Constantes del control auxiliar

%minimize sigma
alpha = [5; 5; 0.5; 5; 5; 10];

%aumetnar control, aumentar energía del sistema
beta = [0.5; 0.5; 7.5; 0.05; 0.05; 5];

%% ine, solicitud, toelf ibt, carta promedio

== matlab function hexa_tilted_ANSFT/Constants Functions ==
  data: Phi output; R1 output; Rib output; Fg output; pose input; M output; M_inv output; allo output; v input
function [Phi, R1, Rib, Fg, M, M_inv, allo] = fcn(pose, v)

%% system constants
pi = 3.141592;
m = 2.0; %5 mass 2.2 kg
l = 0.25; % length m
g = 9.81; % gravity m/s²
Jxx =  24778420.82/(1000*1000000); % kg m²
Jyy = 42217933.96/(1000*1000000); % kg m²
Jzz = 23948304.24/(1000*1000000); % kg m²
kT = 0.000006975938113;
kQ = 0.000118290418538;

%% Phi matrix calculation
uu = v(1);
vv = v(2);
ww = v(3);
pp = v(4);
qq = v(5);
rr = v(6);


Phi = [0, -rr, qq, 0, -ww, vv;
        rr, 0, -pp , ww, 0, -uu;
        -qq, pp, 0,  -vv, uu, 0;
        0, 0, 0, 0, -rr, qq; 
        0, 0, 0, rr, 0, -pp;
        0, 0, 0, -qq, pp, 0];

%% Rib matrix calculation

roll = pose(4);
pitch = pose(5);
yaw = pose(6);

R1 = [cos(yaw)*cos(pitch), -cos(roll)*sin(yaw) + cos(yaw)*sin(roll)*sin(pitch), sin(roll)*sin(yaw) + cos(roll)*cos(yaw)*sin(pitch);
       cos(pitch)*sin(yaw), cos(roll)*cos(yaw) + sin(yaw)*sin(pitch)*sin(roll), -cos(yaw)*sin(roll) + sin(yaw)*sin(pitch)*cos(roll);
       -sin(pitch), cos(pitch)*sin(roll), cos(pitch)*cos(roll)];

R2 = [1, sin(roll)*tan(pitch), cos(roll)*tan(pitch);
      0, cos(roll), -sin(roll);
      0, sin(roll)/cos(pitch), cos(roll)/cos(pitch)];

Rzeros = zeros(3);

% Rib = [cos(yaw)*cos(pitch), -cos(roll)*sin(yaw) + cos(yaw)*sin(roll)*sin(pitch), sin(roll)*sin(yaw) + cos(roll)*cos(yaw)*sin(pitch), 0, 0, 0;
%        cos(pitch)*sin(yaw), cos(roll)*cos(yaw) + sin(yaw)*sin(pitch)*sin(roll), -cos(yaw)*sin(roll) + sin(yaw)*sin(pitch)*cos(roll), 0, 0, 0;
%        -sin(pitch), cos(pitch)*sin(roll), cos(pitch)*cos(roll), 0, 0, 0;
%        0, 0, 0, 1, sin(roll)*tan(pitch), cos(roll)*tan(pitch);
%        0, 0, 0, 0, cos(roll), -sin(roll);
%        0, 0, 0, 0, sin(roll)/cos(pitch), cos(roll)/cos(pitch)];

Rib = [R1, Rzeros;
       Rzeros, R2];

%% Fg matrix calculation

Fg = [m*g*sin(pitch);
      -m*g*cos(pitch)*sin(roll);
      -m*g*cos(pitch)*cos(roll);
      0;
      0;
      0];

M = [m, 0, 0, 0, 0, 0;
    0, m, 0, 0, 0, 0;
    0, 0, m, 0, 0, 0;
    0, 0, 0, Jxx, 0, 0;
    0, 0, 0, 0, Jyy, 0;
    0, 0, 0, 0, 0, Jzz];

M_inv = inv(M);

alpha = [pi/6; -pi/6; -pi/2; -5*pi/6; 5*pi/6; pi/2];

varphi = pi/9;

%% tilted rotors matrix allocation

m11 = -kT*cos(alpha(1))*sin(varphi);
m21 = kT*sin(alpha(1))*sin(varphi);
m31 = kT*cos(varphi);
m41 = cos(alpha(1))*(l*kT*cos(varphi) - kQ*sin(varphi));
m51 = sin(alpha(1))*(-l*kT*cos(varphi) + kQ*sin(varphi));
m61 = l*kT*sin(varphi) + kQ*cos(varphi);

m12 = kT*cos(alpha(2))*sin(varphi);
m22 = -kT*sin(alpha(2))*sin(varphi);
m32 = m31;
m42 = cos(alpha(2))*(l*kT*cos(varphi) - kQ*sin(varphi));
m52 = sin(alpha(2))*(-l*kT*cos(varphi) + kQ*sin(varphi));
m62 = -l*kT*sin(varphi) - kQ*cos(varphi);

m13 = kT*cos(alpha(3))*sin(varphi);
m23 = kT*sin(alpha(3))*sin(varphi);
m33 = m31;
m43 = cos(alpha(3))*(l*kT*cos(varphi) + kQ*sin(varphi));
m53 = sin(alpha(3))*(-l*kT*cos(varphi) + kQ*sin(varphi));
m63 = l*kT*sin(varphi) + kQ*cos(varphi);

m14 = kT*cos(alpha(4))*sin(varphi);
m24 = -kT*sin(alpha(4))*sin(varphi);
m34 = m31;
m44 = cos(alpha(4))*(l*kT*cos(varphi) - kQ*sin(varphi));
m54 = sin(alpha(4))*(-l*kT*cos(varphi) + kQ*sin(varphi));
m64 = -l*kT*sin(varphi) - kQ*cos(varphi);

m15 = -kT*cos(alpha(5))*sin(varphi);
m25 = kT*sin(alpha(5))*sin(varphi);
m35 = m31;
m45 = cos(alpha(5))*(l*kT*cos(varphi) - kQ*sin(varphi));
m55 = sin(alpha(5))*(-l*kT*cos(varphi) + kQ*sin(varphi));
m65 = l*kT*sin(varphi) + kQ*cos(varphi);

m16 = kT*cos(alpha(6))*sin(varphi);
m26 = -kT*sin(alpha(6))*sin(varphi);
m36 = m31;
m46 = cos(alpha(6))*(l*kT*cos(varphi) + kQ*sin(varphi));
m56 = sin(alpha(6))*(-l*kT*cos(varphi) + kQ*sin(varphi));
m66 = -l*kT*sin(varphi) - kQ*cos(varphi);

allo = [m11, m12, m13, m14, m15, m16;
        m21, m22, m23, m24, m25, m26;
        m31, m32, m33, m34, m35, m36;
        m41, m42, m43, m44, m45, m46;
        m51, m52, m53, m54, m55, m56;
        m61, m62, m63, m64, m65, m66];

allo = inv(allo);

== matlab function hexa_tilted_ANSFT/Lemniscate Trajectory ==
  data: time input; pose_d output; pose_d_dot output; pose_d_ddot output
function [pose_d, pose_d_dot, pose_d_ddot]= fcn(time)

%% Positions

arg = time / 4;

pos_x = cos(arg) ./ (1 + sin(arg) .* sin(arg));
pos_y = cos(arg) .* sin(arg) ./ (1 + sin(arg) .* sin(arg));
pos_z = time / 12;

yaw = time * 0;

pose_d = [pos_x;
          pos_y;
          pos_z;
          0;
          0;
          yaw];

%% Velocities

pos_z_dot = 1 / 12;
pos_x_dot = 0;
pos_y_dot = 0;
yaw_dot = 0;

pose_d_dot = [pos_x_dot;
              pos_y_dot;
              pos_z_dot;
              0;
              0;
              yaw_dot];

%% Accelerations

pos_z_ddot = 0;
pos_x_ddot = 0;
pos_y_ddot = 0;
yaw_ddot = 0;

pose_d_ddot = [pos_x_ddot;
               pos_y_ddot;
               pos_z_ddot;
               0;
               0;
               yaw_ddot];
